simulink model "homework_4_1"  (R2023a)
settings: Solver=VariableStepAuto  StartTime=0.0  StopTime=10.0  RelTol=1e-3
undefined symbols (not defined in the file): beta, Ce, Te, Tm
settings Model: Creator=matve  LastModifiedBy=matve

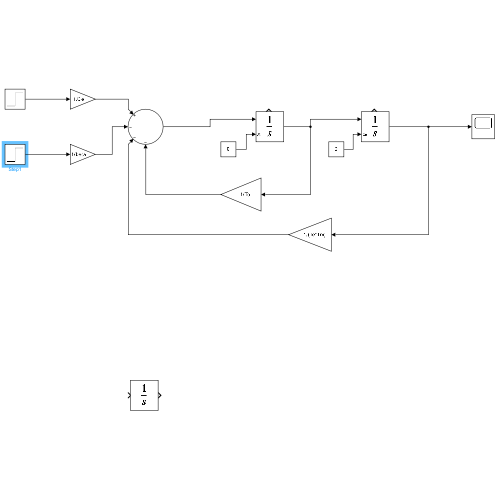
[thumbnail: Simulink's stored preview of the top-level diagram]
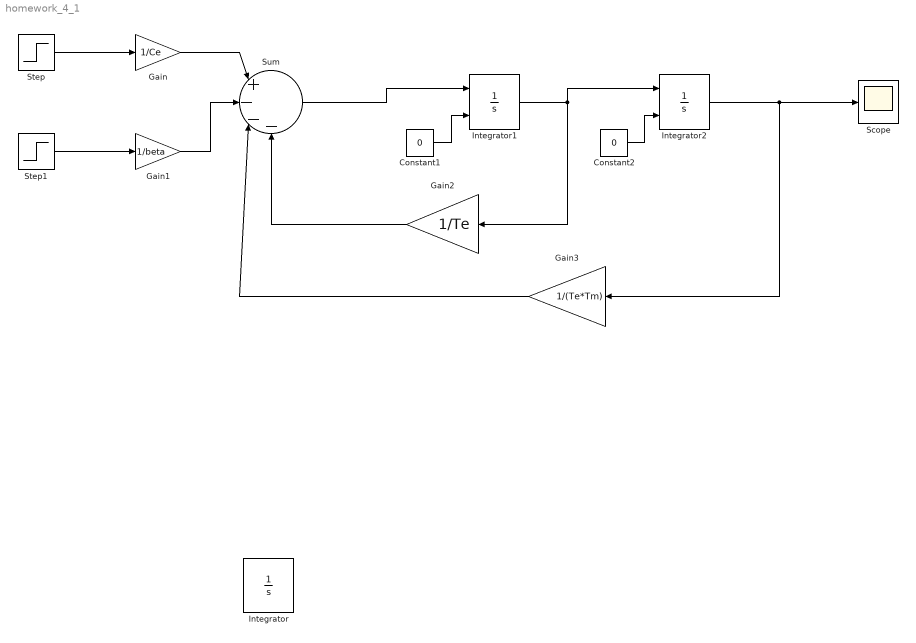
== system homework_4_1 ==
  Constant1 : Constant  Value=0
  Constant2 : Constant  Value=0
  Gain : Gain  Gain=1/Ce
  Gain1 : Gain  Gain=1/beta
  Gain2 : Gain  Gain=1/Te
  Gain3 : Gain  Gain=1/(Te*Tm)
  Integrator : Integrator
  Integrator1 : Integrator  InitialConditionSource=external  ShowStatePort=on
  Integrator2 : Integrator  InitialConditionSource=external  ShowStatePort=on
  Scope : Scope
  Step : Step  SampleTime=0
  Step1 : Step  SampleTime=0
  Sum : Sum  Inputs=|+---
  wires:
  Step/1 -> Gain/1
  Step1/1 -> Gain1/1
  Gain/1 -> Sum/1
  Gain1/1 -> Sum/2
  Sum/1 -> Integrator1/1
  Integrator1/1 -> Integrator2/1, Gain2/1
  Gain2/1 -> Sum/4
  Integrator2/1 -> Gain3/1, Scope/1
  Gain3/1 -> Sum/3
  Constant1/1 -> Integrator1/2
  Constant2/1 -> Integrator2/2
